simulink model "Mega2560Monitoreo"  (R2021b)
settings: Solver=ode2  StartTime=0.0  StopTime=inf  FixedStep=0.009  RelTol=1e-3  EnableMultiTasking=on
undefined symbols (not defined in the file): gv
libraries: arduinolib x10, arduinosensorlib x1
settings Model: SimulationMode=external  ExtModeTrigDuration=2  Creator=Jka  LastModifiedBy=alex_
settings SolverCC: AlgebraicLoopSolver=TrustRegion  AutoInsertRateTranBlk=on
settings OptimizationCC: EnhancedBackFolding=on  PassReuseOutputArgsThreshold=0  MaxStackSize=64  OptimizeBlockOrder=speed  DifferentSizesBufferReuse=on  OptimizationCustomize=off
settings DebuggingCC: ParameterTunabilityLossMsg=error  SFMachineParentedDataDiag=warning
settings HardwareCC: ProdBitPerInt=16  ProdBitPerPointer=16  ProdBitPerSizeT=16  ProdBitPerPtrDiffT=16  ProdLargestAtomicFloat=None  ProdWordSize=8  ProdHWDeviceType=Atmel->AVR  UseEmbeddedCoderFeatures=off  UseSimulinkCoderFeatures=off
settings SFSimCC: MATLABDynamicMemAlloc=off
settings RTWCC: Description=Embedded Coder  SystemTargetFile=ert.tlc  HardwareBoard=Arduino Mega 2560  TemplateMakefile=ert_default_tmf  RTWVerbose=off  Toolchain=Arduino AVR  BuildConfiguration=Faster Runs
settings CodeAppCC: ForceParamTrailComments=on  OperatorAnnotations=on  MangleLength=10
settings ERTTargetCC: ERTCustomFileBanners=off  SupportContinuousTime=on  SupportNonInlinedSFcns=on  RemoveResetFunc=off  SupportVariableSizeSignals=on  ModelStepFunctionPrototypeControlCompliant=off  ExtMode=on  ExtModeTransport=3  ExtModeStaticAlloc=on  ExtModeStaticAllocSize=2048  ExtModeMexFile=ext_xcp  ExtModeMexArgs=1 3 921600  ExtModeIntrfLevel=Level2 - Open  ERTSrcFileBannerTemplate=codertarget_code_template.cgt  ERTHdrFileBannerTemplate=codertarget_code_template.cgt  ERTDataSrcFileTemplate=codertarget_code_template.cgt  ERTDataHdrFileTemplate=codertarget_code_template.cgt

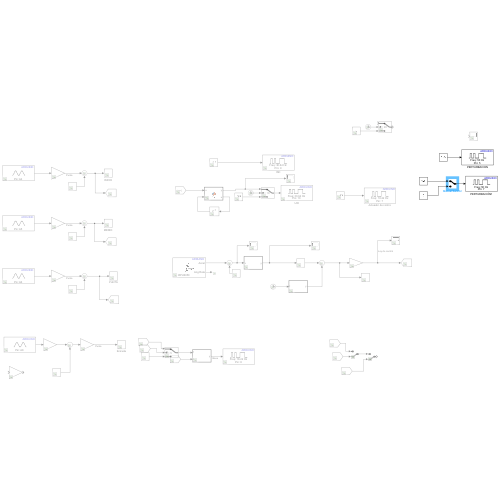
[thumbnail: Simulink's stored preview of the top-level diagram]
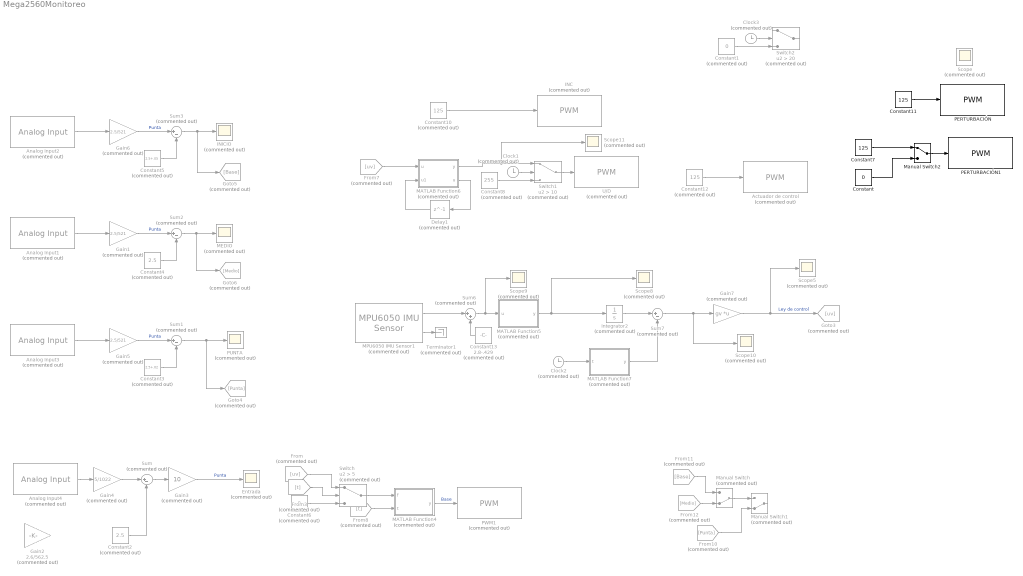
== system Mega2560Monitoreo ==
  Actuador de control : arduinolib/PWM  Commented=on  pinNumber=7  frequencyType=Specify  desiredFrequency=w1  achievableFrequency=18.2186
  Analog Input1 : arduinolib/Analog Input  Commented=on  pinNumber=5  ReadResultsOnly=off  ConversionTriggerSource=Software  ExternalTriggerType=uint32( 0 )  OutputDataType=uint16  EnableConversionCompleteNotify=off  EnableOuputStatus=off  SampleTime=-1  blockPlatform=arduino
  Analog Input2 : arduinolib/Analog Input  Commented=on  pinNumber=4  ReadResultsOnly=off  ConversionTriggerSource=Software  ExternalTriggerType=uint32( 0 )  OutputDataType=uint16  EnableConversionCompleteNotify=off  EnableOuputStatus=off  SampleTime=-1  blockPlatform=arduino
  Analog Input3 : arduinolib/Analog Input  Commented=on  pinNumber=6  ReadResultsOnly=off  ConversionTriggerSource=Software  ExternalTriggerType=uint32( 0 )  OutputDataType=uint16  EnableConversionCompleteNotify=off  EnableOuputStatus=off  SampleTime=-1  blockPlatform=arduino
  Analog Input4 : arduinolib/Analog Input  Commented=on  pinNumber=8  ReadResultsOnly=off  ConversionTriggerSource=Software  ExternalTriggerType=uint32( 0 )  OutputDataType=uint16  EnableConversionCompleteNotify=off  EnableOuputStatus=off  SampleTime=-1  blockPlatform=arduino
  Clock1 : Clock  Commented=on
  Clock2 : Clock  Commented=on
  Clock3 : Clock  Commented=on
  Constant : Constant  Value=0
  Constant1 : Constant  Commented=on  Value=0
  Constant10 : Constant  Commented=on  Value=125
  Constant11 : Constant  Value=125
  Constant12 : Constant  Commented=on  Value=125
  Constant13 : Constant  Commented=on  Value=2.8-.429
  Constant2 : Constant  Commented=on  Value=2.5
  Constant3 : Constant  Commented=on  Value=2.5+.02
  Constant4 : Constant  Commented=on  Value=2.5
  Constant5 : Constant  Commented=on  Value=2.5+.05
  Constant6 : Constant  Commented=on  Value=0
  Constant7 : Constant  Value=125
  Constant8 : Constant  Commented=on  Value=255
  Delay1 : Delay  Commented=on  DelayLength=1
  Entrada : Scope  Commented=on
  From : From  Commented=on  GotoTag=uv
  From10 : From  Commented=on  GotoTag=Punta
  From11 : From  Commented=on  GotoTag=Base
  From12 : From  Commented=on  GotoTag=Medio
  From3 : From  Commented=on  GotoTag=t
  From7 : From  Commented=on  GotoTag=uv
  From8 : From  Commented=on  GotoTag=t
  Gain1 : Gain  Commented=on  Gain=2.5/521
  Gain2 : Gain  Commented=on  Gain=2.6/562.5
  Gain3 : Gain  Commented=on  Gain=10
  Gain4 : Gain  Commented=on  Gain=5/1022
  Gain5 : Gain  Commented=on  Gain=2.5/521
  Gain6 : Gain  Commented=on  Gain=2.5/521
  Gain7 : Gain  Commented=on  Gain=gv  Multiplication=Matrix(K*u)
  Goto3 : Goto  Commented=on  GotoTag=uv
  Goto4 : Goto  Commented=on  GotoTag=Punta
  Goto5 : Goto  Commented=on  GotoTag=Base
  Goto6 : Goto  Commented=on  GotoTag=Medio
  INC : arduinolib/PWM  Commented=on  pinNumber=9  frequencyType=Specify  desiredFrequency=30.64  achievableFrequency=30.64
  INICIO : Scope  Commented=on
  Integrator2 : Integrator  Commented=on  UpperSaturationLimit=5  LowerSaturationLimit=-5
  MATLAB Function4 : MATLAB Function  Commented=on  TreatAsAtomicUnit=on
  MATLAB Function5 : MATLAB Function  Commented=on  TreatAsAtomicUnit=on
  MATLAB Function6 : MATLAB Function  Commented=on  TreatAsAtomicUnit=on
  MATLAB Function7 : MATLAB Function  Commented=on  TreatAsAtomicUnit=on
  MEDIO : Scope  Commented=on
  MPU6050 IMU Sensor1 : arduinosensorlib/MPU6050 IMU Sensor  Commented=on  SlaveAddress=0x68  Accel=on  AngularRate=on  Temperature=off  Status=off  EulerAngles=off  Quat=off  AccelRange=2G  GyroRange=250 dps  DmpOdr=200 Hz  Dlpf=Accelerometer: 184Hz, Gyroscope: 188Hz  SampleTime=-1
      settings: SourceProductBaseCode=ARDUINO
  Manual Switch : ManualSwitch  Commented=on  CurrentSetting=0
  Manual Switch1 : ManualSwitch  Commented=on  CurrentSetting=0
  Manual Switch2 : ManualSwitch
  PERTURBACIÓN : arduinolib/PWM  pinNumber=5  frequencyType=Specify  desiredFrequency=50  achievableFrequency=50
  PERTURBACIÓN1 : arduinolib/PWM  pinNumber=7  frequencyType=Specify  desiredFrequency=50  achievableFrequency=50
  PUNTA : Scope  Commented=on
  PWM1 : arduinolib/PWM  Commented=on  pinNumber=8  frequencyType=Specify  desiredFrequency=w1  achievableFrequency=18.2186
  Scope{,5,8..11} (6 alike) : Scope  Commented=on
  Sum{,1..3,7} (5 alike) : Sum  Commented=on  Inputs=|+-
  Sum6 : Sum  Commented=on  Inputs=|++
  Switch : Switch  Commented=on  Criteria=u2 > Threshold  Threshold=5
  Switch1 : Switch  Commented=on  Criteria=u2 > Threshold  Threshold=10
  Switch2 : Switch  Commented=on  Criteria=u2 > Threshold  Threshold=20
  Terminator1 : Terminator  Commented=on
  U/D : arduinolib/PWM  Commented=on  pinNumber=10  frequencyType=Specify  desiredFrequency=30.64  achievableFrequency=30.64
  wires:
  Analog Input2/1 -> Gain6/1
  Analog Input1/1 -> Gain1/1
  Analog Input3/1 -> Gain5/1
  From8/1 -> MATLAB Function4/2(t)
  Constant2/1 -> Sum/2
  Gain3/1 -> Entrada/1  "Punta"
  Analog Input4/1 -> Gain4/1
  Gain4/1 -> Sum/1
  Sum/1 -> Gain3/1
  Gain5/1 -> Sum1/1  "Punta"
  Sum1/1 -> Goto4/1, PUNTA/1
  Constant3/1 -> Sum1/2
  Sum2/1 -> Goto6/1, MEDIO/1
  Gain1/1 -> Sum2/1  "Punta"
  Constant4/1 -> Sum2/2
  Sum3/1 -> Goto5/1, INICIO/1
  Gain6/1 -> Sum3/1  "Punta"
  Constant5/1 -> Sum3/2
  From3/1 -> Switch/2
  Constant6/1 -> Switch/3
  From/1 -> Switch/1
  MATLAB Function4/1(y) -> PWM1/1  "Base"
  Switch/1 -> MATLAB Function4/1(f)
  Constant8/1 -> Switch1/3
  Constant10/1 -> INC/1
  Constant12/1 -> Actuador de control/1
  Gain7/1 -> Goto3/1, Scope5/1  "Ley de control"
  MATLAB Function5/1(y) -> Scope8/1, Integrator2/1
  MPU6050 IMU Sensor1/1 -> Sum6/1
  MPU6050 IMU Sensor1/2 -> Terminator1/1
  Sum6/1 -> Scope9/1, MATLAB Function5/1(u)
  Constant13/1 -> Sum6/2
  Clock1/1 -> Switch1/2
  Delay1/1 -> MATLAB Function6/2(u1)
  MATLAB Function6/2(u) -> Delay1/1
  From7/1 -> MATLAB Function6/1("u ")
  Switch1/1 -> U/D/1
  MATLAB Function6/1(y) -> Scope11/1, Switch1/1
  Integrator2/1 -> Sum7/1
  MATLAB Function7/1(y) -> Sum7/2
  Clock2/1 -> MATLAB Function7/1(t)
  Manual Switch/1 -> Manual Switch1/1
  From10/1 -> Manual Switch1/2
  From11/1 -> Manual Switch/1
  From12/1 -> Manual Switch/2
  Sum7/1 -> Scope10/1, Gain7/1
  Clock3/1 -> Switch2/2
  Constant1/1 -> Switch2/3
  Constant11/1 -> PERTURBACIÓN/1
  Constant7/1 -> Manual Switch2/1
  Constant/1 -> Manual Switch2/2
  Manual Switch2/1 -> PERTURBACIÓN1/1

== matlab function Mega2560Monitoreo/MATLAB Function4 ==
  data: f input; t input; y output
function y = fcn(f,t)



% f=120*(sin(t)+3.18);
% f=30;%frecuencia

%recordar que si para manipular f necesito t entonces y no debe tener t
% de lo contrario existirìa un t al cuadrado
y=128*(square(2*pi*f*t,50)+1);
end

== matlab function Mega2560Monitoreo/MATLAB Function5 ==
  data: u input; y output
function y = fcn(u)

x = u(3,:,:);
a=0.04;
if x<a && x>-a
    y=0;
else
    y=x;
end

== matlab function Mega2560Monitoreo/MATLAB Function6 ==
  data: u input; y output; u output; u1 input
function [y,u] = fcn(u,u1)

k1=u;
k2=u1;
    
if k1>k2
    y=1;
else 
    y=0;
end
end

== matlab function Mega2560Monitoreo/MATLAB Function7 ==
  data: t input; y output
function y = fcn(t)

m=0.2846;

y = m*t;
